simulink model "EEE463_HardwareProject_w_Real_Components"  (R2024b)
settings: Solver=VariableStepAuto  StartTime=0.0  StopTime=5  RelTol=1e-3
libraries: spsDiodeLib x7, spsCurrentMeasurementLib x5, spsVoltageMeasurementLib x5, spsSeriesRLCBranchLib x3, spsDCMachineLib x1, spsDCVoltageSourceLib x1, spsGroundLib x1, spsMosfetLib x1, spsThreePhaseProgrammableVoltageSourceLib x1, spsThreePhaseVIMeasurementLib x1, sps_lib x1
settings Model: Creator=Asus  LastModifiedBy=Asus

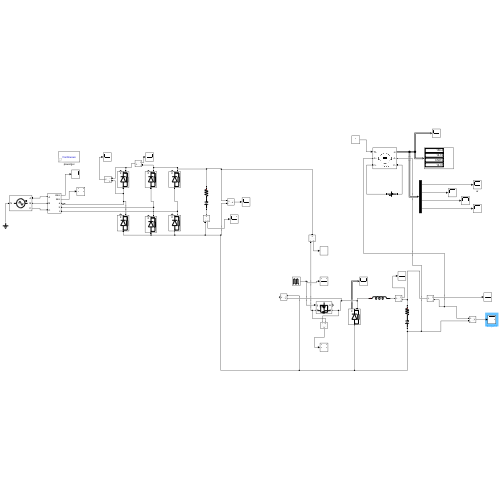
[thumbnail: Simulink's stored preview of the top-level diagram]
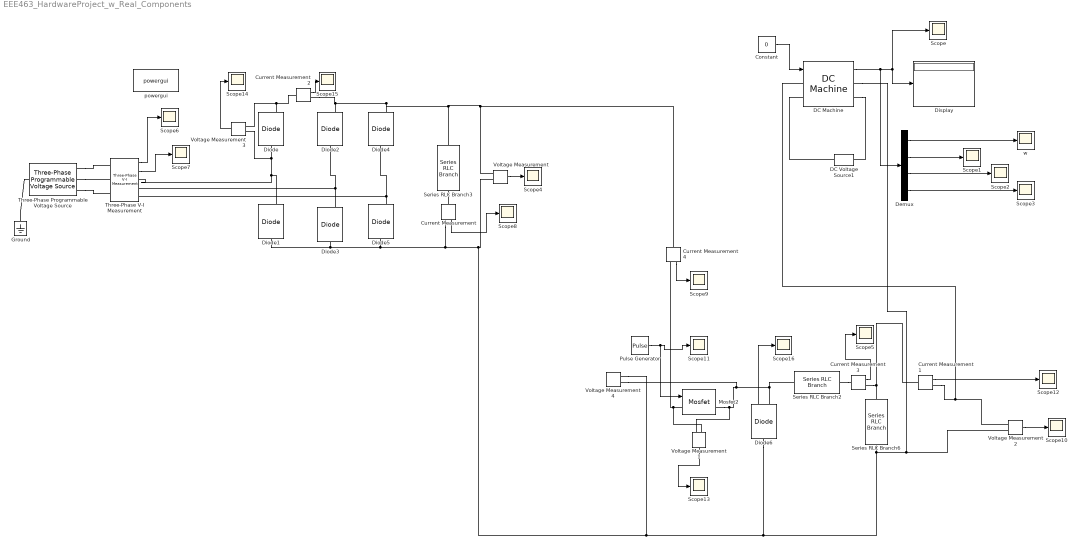
== system EEE463_HardwareProject_w_Real_Components ==
  Constant : Constant  Value=0
  Current Measurement{,1..4} (5 alike) : spsCurrentMeasurementLib/Current Measurement  PhasorSimulation=off  OutputType=Complex  PSBequivalent=0
  DC Machine : spsDCMachineLib/DC Machine  PresetModel=No  MechanicalLoad=Torque TL  FieldType=Wound  ShowDetailedParameters=on  MeasurementBus=off  RLa="[ 0.8  0.0125]"  RLf="[ 210  23]"  Laf=1.8  MachineConstant=Torque constant (N.m/A)  Ke=1.8  Kt=1.8  J=1  Bm=0.1  Tf=0.1  w0=1  Ifinit=0.561904761878152  TsPowergui=0  TsBlock=-1
  DC Voltage Source1 : spsDCVoltageSourceLib/DC Voltage Source  Amplitude=118  Measurements=None
  Demux : Demux
  Diode{,1..5} (6 alike) : spsDiodeLib/Diode  Ron=0.0325  Lon=0  Vf=0.98  IC=0  UseSnubber=0  Rs=500  Cs=250e-9  Measurements=on
  Diode6 : spsDiodeLib/Diode  Ron=0.217  Lon=0  Vf=1.3  IC=0  UseSnubber=0  Rs=500  Cs=250e-9  Measurements=on
  Display : Display
  Ground : spsGroundLib/Ground  LConnTagsString=a
  Mosfet2 : spsMosfetLib/Mosfet  Ron=0.1  Lon=0  Rd=0.01  Vfd=0  IC=0  Rs=1e5  Cs=inf  Measurements=on
  Pulse Generator : DiscretePulseGenerator  PulseType=Time based  Amplitude=5  Period=1/10000  PulseWidth=85
  Scope{,1..16} (17 alike) : Scope
  Series RLC Branch2 : spsSeriesRLCBranchLib/Series RLC Branch  LConnTagsString=__new0  RConnTagsString=__new0  BranchType=L  Resistance=1  Inductance=230e-6  SetiL0=off  InitialCurrent=0  Capacitance=1e-6  Setx0=off  InitialVoltage=0  Measurements=None
  Series RLC Branch3 : spsSeriesRLCBranchLib/Series RLC Branch  LConnTagsString=__new0  RConnTagsString=__new0  BranchType=RC  Resistance=0.04  Inductance=1e-3  SetiL0=off  InitialCurrent=0  Capacitance=1000e-6  Setx0=off  InitialVoltage=0  Measurements=None
  Series RLC Branch6 : spsSeriesRLCBranchLib/Series RLC Branch  LConnTagsString=__new0  RConnTagsString=__new0  BranchType=RC  Resistance=0.03  Inductance=1e-3  SetiL0=off  InitialCurrent=0  Capacitance=680e-6  Setx0=off  InitialVoltage=0  Measurements=None
  Three-Phase Programmable Voltage Source : spsThreePhaseProgrammableVoltageSourceLib/Three-Phase Programmable Voltage Source  PositiveSequence="[150  0 50]"  VariationEntity=None  VariationType=Table of time-amplitude pairs  VariationTypeAlt=Step  VariationStep=0.5  VariationRate=10  VariationMagnitude=0.3  VariationFrequency=2  VariationTiming=[1 2]  VariationPhaseA=off  Amplitudes="[0.1  0.3  0.5  0.7  0.9 1]"  TimeValues="[0  0.2  0.4  0.6  0.8 0.9]"  HarmonicGeneration=off  HarmonicA=[3 0.2 -25 0]  HarmonicB=[2 0.15 35 2]  Timing="[0.05  3]"  BusType=swing  Pref=0  Qref=0  Qmin=-inf  Qmax=inf
  Three-Phase V-I Measurement : spsThreePhaseVIMeasurementLib/Three-Phase V-I Measurement  VoltageMeasurement=phase-to-phase  SetLabelV=off  LabelV=Vabc  Vpu=off  VpuLL=off  CurrentMeasurement=yes  SetLabelI=off  LabelI=Iabc  Ipu=off  Pbase=100e6  Vbase=500e3  OutputType=Complex  PhasorSimulation=off  PSBequivalent=0
  Voltage Measurement{,1..4} (5 alike) : spsVoltageMeasurementLib/Voltage Measurement  PhasorSimulation=off  OutputType=Complex  PSBequivalent=0
  powergui : sps_lib/powergui  Priority=1  SimulationMode=Continuous  SampleTime=50e-6  frequency=60  Iterations=50  frequencyindice=0  Pbase=100e6  ErrMax=1e-4  UnitsV=kV  UnitsW=MW  buscounter=0  FunctionMessages=off  echomessages=off  EnableUseOfTLC=off  CurrentSourceSwitches=off  DisableSnubberDevices=off  DisableRonSwitches=off  DisableVfSwitches=off  DisplayEquations=off  AutomaticDiscreteSolvers=off  SolverType=Tustin/Backward Euler (TBE)  Interpol=off  ExternalGateDelay=off  methode=off  Ts=100  x0status=blocks  SPID=on  SwTol=0  HookPort=off  NonlinearTolerance=1e-4  nMaxIteration=100  ContinueOnMaxIteration=off  RestoreLinks=warning  ResistiveCurrentMeasurement=off  Frange=[0:2:500]  Ylog=off  Xlog=on  ShowGrid=off  save=off  variable=ZData  structure=0  ZoomFFT=off  StartTime=0.0  cycles=1  DisplayStyle=1  fundamental=60  FreqAxis=off  MaxFrequency=1000  frequencyindicesteady=1  RmsSteady=1  display=off
  w : Scope
  wires:
  Three-Phase V-I Measurement/1 -> Scope6/1
  Voltage Measurement/1 -> Scope4/1
  Current Measurement/1 -> Scope8/1
  Three-Phase V-I Measurement/2 -> Scope7/1
  Current Measurement2/1 -> Scope15/1
  DC Machine/1 -> Demux/1, Scope/1, Display/1
  Voltage Measurement2/1 -> Scope10/1
  Demux/2 -> Scope1/1
  Demux/4 -> Scope3/1
  Current Measurement1/1 -> Scope12/1
  Constant/1 -> DC Machine/1
  Pulse Generator/1 -> Scope11/1, Mosfet2/1
  Demux/3 -> Scope2/1
  Demux/1 -> w/1
  Current Measurement3/1 -> Scope5/1
  Current Measurement4/1 -> Scope9/1
  Voltage Measurement1/1 -> Scope13/1
  Voltage Measurement3/1 -> Scope14/1
  Diode6/1 -> Scope16/1
  connections:
  Diode4/RConn1 -- Current Measurement4/LConn1 -- Voltage Measurement/LConn1 -- Series RLC Branch3/LConn1 -- Current Measurement2/RConn1 -- Diode2/RConn1
  Diode6/LConn1 -- Voltage Measurement2/LConn2 -- DC Machine/RConn1 -- Series RLC Branch6/RConn1 -- Voltage Measurement4/LConn2 -- Current Measurement/RConn1 -- Diode5/LConn1 -- Diode1/LConn1 -- Diode3/LConn1 -- Voltage Measurement/LConn2
  Diode1/RConn1 -- Three-Phase V-I Measurement/RConn1 -- Voltage Measurement3/LConn1 -- Diode/LConn1
  Diode2/LConn1 -- Diode3/RConn1 -- Three-Phase V-I Measurement/RConn2
  Diode4/LConn1 -- Diode5/RConn1 -- Three-Phase V-I Measurement/RConn3
  Diode/RConn1 -- Voltage Measurement3/LConn2 -- Current Measurement2/LConn1
  Three-Phase Programmable Voltage Source/RConn2 -- Three-Phase V-I Measurement/LConn2
  Ground/LConn1 -- Three-Phase Programmable Voltage Source/LConn1
  Three-Phase Programmable Voltage Source/RConn1 -- Three-Phase V-I Measurement/LConn1
  Current Measurement/LConn1 -- Series RLC Branch3/RConn1
  Three-Phase Programmable Voltage Source/RConn3 -- Three-Phase V-I Measurement/LConn3
  Diode6/RConn1 -- Voltage Measurement4/LConn1 -- Voltage Measurement1/LConn2 -- Mosfet2/RConn1 -- Series RLC Branch2/LConn1
  Current Measurement1/LConn1 -- Current Measurement3/RConn1 -- Series RLC Branch6/LConn1
  Voltage Measurement2/LConn1 -- Current Measurement1/RConn1 -- DC Machine/LConn1
  DC Voltage Source1/RConn1 -- DC Machine/LConn2
  DC Machine/RConn2 -- DC Voltage Source1/LConn1
  Series RLC Branch2/RConn1 -- Current Measurement3/LConn1
  Mosfet2/LConn1 -- Voltage Measurement1/LConn1 -- Current Measurement4/RConn1
